simulink model "example_LineFollowerAnalogInput"  (Simulink 7.0)
settings: Solver=FixedStepDiscrete  StartTime=0.0  StopTime=inf  FixedStep=20  RelTol=1e-3
libraries: lib_robotinohardware x6
settings Model: Creator=indorewala  LastModifiedBy=indorewala

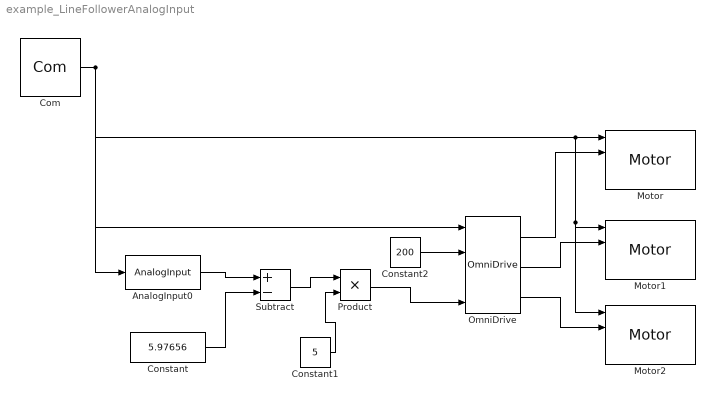
== system example_LineFollowerAnalogInput ==
  AnalogInput0 : lib_robotinohardware/AnalogInput  num=0
  Com : lib_robotinohardware/Com  ip='127.0.0.1'
  Constant : Constant  Value=5.97656  OutDataType=sfix(16)  OutScaling=2^0
  Constant1 : Constant  Value=5  OutDataType=sfix(16)  OutScaling=2^0
  Constant2 : Constant  Value=200  OutDataType=sfix(16)  OutScaling=2^0
  Motor : lib_robotinohardware/Motor  num=0  kp=255  ki=255  kd=255
  Motor1 : lib_robotinohardware/Motor  num=1  kp=255  ki=255  kd=255
  Motor2 : lib_robotinohardware/Motor  num=2  kp=255  ki=255  kd=255
  OmniDrive : lib_robotinohardware/OmniDrive
  Product : Product  OutDataType=sfix(16)  OutScaling=2^0  RndMeth=Zero
  Subtract : Sum  Inputs=+-  OutDataType=sfix(16)  OutScaling=2^-10
  wires:
  Com/1 -> AnalogInput0/1, OmniDrive/1, Motor/1, Motor1/1, Motor2/1
  AnalogInput0/1 -> Subtract/1
  Constant/1 -> Subtract/2
  Subtract/1 -> Product/1
  Constant1/1 -> Product/2
  Product/1 -> OmniDrive/4
  Constant2/1 -> OmniDrive/2
  OmniDrive/1 -> Motor/2
  OmniDrive/2 -> Motor1/2
  OmniDrive/3 -> Motor2/2
